simulink model "AeroPlantMIACpart3"  (Simulink 6.3)
settings: Solver=ode45  StartTime=0.0  StopTime=Tend  RelTol=1e-3
values from neighbouring files (symbols this model uses):
  sigma2e = 0.0    (= 0)    [InitEx5.m]
  Ta = 0.1    [InitEx5.m]
  Tc = 0.01    [InitEx5.m]
  w1 = 1    [InitEx5.m]    (also in SynthesisEx5.m = 0)
  w2 = 1    [InitEx5.m]    (also in SynthesisEx5.m = 0)
  w3 = 1    [InitEx5.m]    (also in SynthesisEx5.m = 0)
  wr = 0.5    [InitEx5.m]
  Yr = 1    [InitEx5.m]
libraries: simulink x3
settings Model: LastModifiedBy=Laboratorium

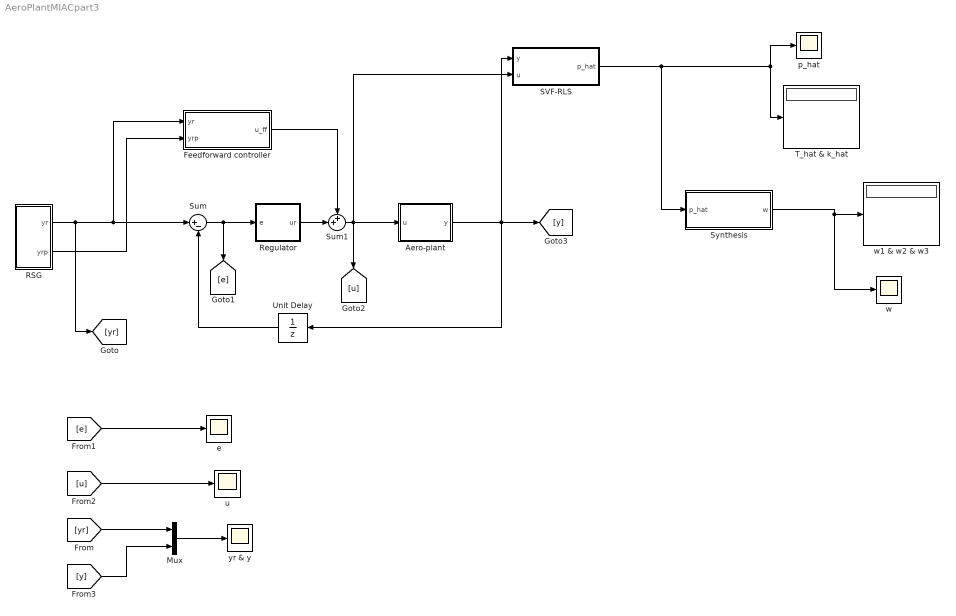
== system AeroPlantMIACpart3 ==
  Aero-plant : Subsystem
  Feedforward controller : Subsystem
  Mux : Mux  Inputs=2
  RSG : Subsystem
  Regulator : Subsystem
  SVF-RLS : Subsystem
  Sum : Sum  Inputs=|+-
  Sum1 : Sum  Inputs=++|
  Synthesis : Subsystem
  T_hat & k_hat : Display
  Unit Delay : UnitDelay  Orientation=left  SampleTime=Tc
  e : Scope
      settings: SaveName=ScopeData6
  p_hat : Scope
      settings: SaveName=ScopeData3
  u : Scope
      settings: SaveName=ScopeData4
  w : Scope
      settings: SaveName=ScopeData2
  w1 & w2 & w3 : Display
  yr & y : Scope
      settings: SaveName=ScopeData5
  wires:
  RSG/1(yr) -> Sum/1, Feedforward controller/1(yr), [yr]
  RSG/2(yrp) -> Feedforward controller/2(yrp)
  SVF-RLS/1(p_hat) -> T_hat & k_hat/1, p_hat/1, Synthesis/1(p_hat)
  Synthesis/1(w) -> w1 & w2 & w3/1, w/1
  Unit Delay/1 -> Sum/2
  Sum/1 -> Regulator/1(e), [e]
  Feedforward controller/1(u_ff) -> Sum1/1
  Regulator/1(ur) -> Sum1/2
  Sum1/1 -> Aero-plant/1(u), SVF-RLS/2(u), [u]
  [yr] -> Mux/1
  [e] -> e/1
  [u] -> u/1
  [y] -> Mux/2
  Mux/1 -> yr & y/1
  Aero-plant/1(y) -> SVF-RLS/1(y), [y], Unit Delay/1

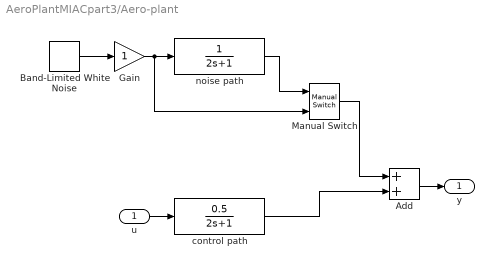
== system AeroPlantMIACpart3/Aero-plant ==
  u : Inport
  Add : Sum  OutScaling=2^-10
  Band-Limited White Noise : simulink/Sources/Band-Limited White Noise  Cov=[sigma2e*Tc]  Ts=Tc  seed=[23341]
  Gain : Gain
  Manual Switch : simulink/Signal Routing/Manual Switch  sw=1  action=0
  control path : TransferFcn  Numerator=[0.5]  Denominator=[2 1]
  noise path : TransferFcn  Denominator=[2 1]
  y : Outport
  wires:
  control path/1 -> Add/2
  Band-Limited White Noise/1 -> Gain/1
  Gain/1 -> Manual Switch/2, noise path/1
  Add/1 -> y/1
  u/1 -> control path/1
  noise path/1 -> Manual Switch/1
  Manual Switch/1 -> Add/1

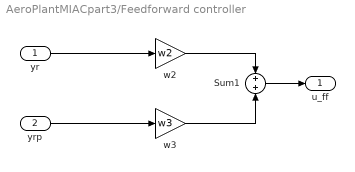
== system AeroPlantMIACpart3/Feedforward controller ==
  yr : Inport
  yrp : Inport  Port=2
  Sum1 : Sum
  w2 : Gain  Gain=w2  SampleTime=Tc
  w3 : Gain  Gain=w3  SampleTime=Tc
  u_ff : Outport
  wires:
  yr/1 -> w2/1
  yrp/1 -> w3/1
  w2/1 -> Sum1/1
  w3/1 -> Sum1/2
  Sum1/1 -> u_ff/1

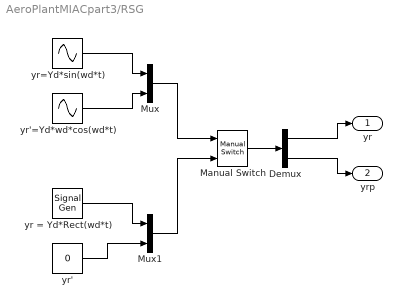
== system AeroPlantMIACpart3/RSG ==
  Demux : Demux  Outputs=2
  Manual Switch : simulink/Signal Routing/Manual Switch  sw=1  action=0
  Mux : Mux  Inputs=2
  Mux1 : Mux  Inputs=2
  yr = Yd*Rect(wd*t) : SignalGenerator  WaveForm=square  Amplitude=Yr  Frequency=wr  Units=rad/sec
  yr' : Constant  Value=0
  yr'=Yd*wd*cos(wd*t) : Sin  Amplitude=Yr*wr  Frequency=wr  Phase=pi/2  SampleTime=0
  yr=Yd*sin(wd*t) : Sin  Amplitude=Yr  Frequency=wr  SampleTime=0
  yr : Outport
  yrp : Outport  Port=2
  wires:
  yr=Yd*sin(wd*t)/1 -> Mux/1
  yr'=Yd*wd*cos(wd*t)/1 -> Mux/2
  yr = Yd*Rect(wd*t)/1 -> Mux1/1
  yr'/1 -> Mux1/2
  Mux/1 -> Manual Switch/1
  Mux1/1 -> Manual Switch/2
  Manual Switch/1 -> Demux/1
  Demux/1 -> yr/1
  Demux/2 -> yrp/1

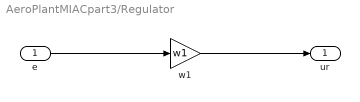
== system AeroPlantMIACpart3/Regulator ==
  e : Inport
  w1 : Gain  Gain=w1  SampleTime=Tc
  ur : Outport
  wires:
  e/1 -> w1/1
  w1/1 -> ur/1

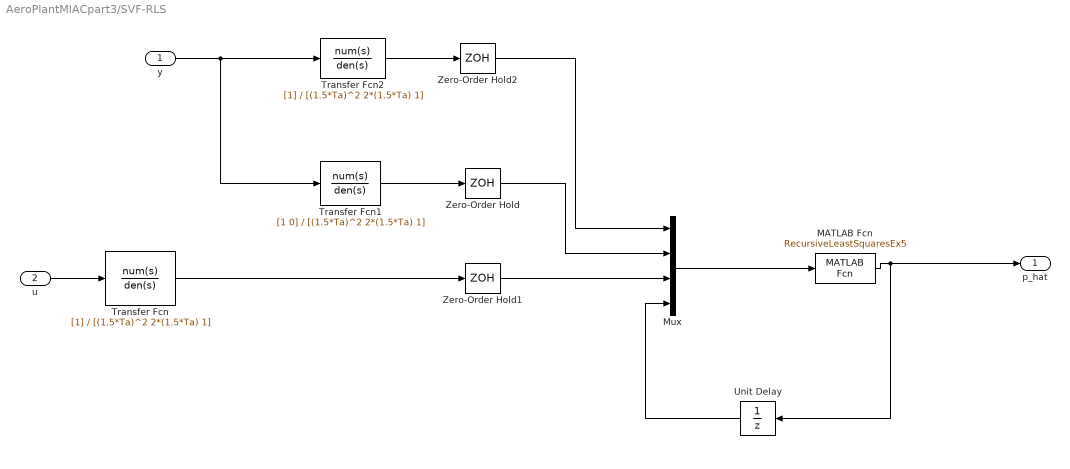
== system AeroPlantMIACpart3/SVF-RLS ==
  y : Inport
  u : Inport  Port=2
  MATLAB Fcn : MATLABFcn  MATLABFcn=RecursiveLeastSquaresEx5  SampleTime=Ta
  Mux : Mux
  Transfer Fcn : TransferFcn  Denominator=[(1.5*Ta)^2 2*(1.5*Ta) 1]
  Transfer Fcn1 : TransferFcn  Numerator=[1 0]  Denominator=[(1.5*Ta)^2 2*(1.5*Ta) 1]
  Transfer Fcn2 : TransferFcn  Denominator=[(1.5*Ta)^2 2*(1.5*Ta) 1]
  Unit Delay : UnitDelay  Orientation=left  SampleTime=Ta
  Zero-Order Hold : ZeroOrderHold  SampleTime=Ta
  Zero-Order Hold1 : ZeroOrderHold  SampleTime=Ta
  Zero-Order Hold2 : ZeroOrderHold  SampleTime=Ta
  p_hat : Outport
  wires:
  Transfer Fcn/1 -> Zero-Order Hold1/1
  Transfer Fcn1/1 -> Zero-Order Hold/1
  Transfer Fcn2/1 -> Zero-Order Hold2/1
  Zero-Order Hold2/1 -> Mux/1
  Zero-Order Hold/1 -> Mux/2
  Zero-Order Hold1/1 -> Mux/3
  Mux/1 -> MATLAB Fcn/1
  MATLAB Fcn/1 -> Unit Delay/1, p_hat/1
  Unit Delay/1 -> Mux/4
  u/1 -> Transfer Fcn/1
  y/1 -> Transfer Fcn2/1, Transfer Fcn1/1

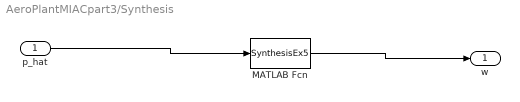
== system AeroPlantMIACpart3/Synthesis ==
  p_hat : Inport
  MATLAB Fcn : MATLABFcn  MATLABFcn=SynthesisEx5  SampleTime=Ta
  w : Outport
  wires:
  p_hat/1 -> MATLAB Fcn/1
  MATLAB Fcn/1 -> w/1
